simulink model "Experiment_cs"  (Simulink 8.8)
settings: Solver=ode5  StartTime=0.0  StopTime=inf  FixedStep=0.0005  RelTol=1e-3
PreLoadFcn:
  | check_NUTS_defined;
  | 
  | assignin('base',['model_closed_' bdroot],false);
InitFcn:
  | PreScanExperimentInitFcn(bdroot)
StopFcn:
  | PreScanExperimentStopFcn(bdroot)
undefined symbols (not defined in the file): DiscIntNeverNeededParam, FromPrescan, IdealSensors, psi, vd01, vd02, vd03, vd04, x, y
libraries: PreScanSimulinkLibrary x12, PreScanUsefulBlocks x8
(part 5 of 5)

== matlab function Toyota_Yaris_1/Dynamics_UserSpecified/SingleVehicle_01/Controller/CtlMainBusUnitDelayAndInit/MATLAB Function ==
  data: u input double; y output Bus: ControllerMainBus; veh_struct parameter double
function y = DelayAndInitCtlBus(u, veh_struct)
coder.extrinsic('exist')
persistent a

y0 = struct;

y0.ActuationCmdBus = struct;
y0.ActuationCmdBus.steering_cmd = 0;
y0.ActuationCmdBus.decel_cmd = 0;
y0.ActuationCmdBus.accel_cmd = 0;

y0.ArbitratedActuationReq = struct;
y0.ArbitratedActuationReq.v_des = 0;
y0.ArbitratedActuationReq.a_des = 0;
y0.ArbitratedActuationReq.psi_des = 0;
y0.ArbitratedActuationReq.dpsi_des = 0;


y0.FunctionFeatures = struct;
y0.FunctionFeatures.wpFollower = struct;
y0.FunctionFeatures.wpFollower.v_des = 0;
y0.FunctionFeatures.wpFollower.a_des = 0;
y0.FunctionFeatures.wpFollower.psi_des = 0;
y0.FunctionFeatures.wpFollower.dpsi_des = 0;


y0.situationBus = struct;
y0.situationBus.wP = struct;

y0.situationBus.wP.finalWayPoint = struct;
y0.situationBus.wP.finalWayPoint.x = 0;
y0.situationBus.wP.finalWayPoint.y = 0;
y0.situationBus.wP.finalWayPoint.z = 0;
y0.situationBus.wP.finalWayPoint.treach = 0;

y0.situationBus.wP.currentWayPoint = struct;
y0.situationBus.wP.currentWayPoint.x = 0;
y0.situationBus.wP.currentWayPoint.y = 0;
y0.situationBus.wP.currentWayPoint.z = 0;
y0.situationBus.wP.currentWayPoint.treach = 0;

y0.situationBus.wP.finalWayPointIndex = uint16(1);
y0.situationBus.wP.currentWayPointIndex = uint16(10);

%y0.situationBus.wP.wayPointArray = struct;
wPArray = struct;
wPArray.x = 0;
wPArray.y = 0;
wPArray.z = 0;
wPArray.treach = 0;
y0.situationBus.wP.wayPointArray = repmat(wPArray,100,1);


y0.situationBus.selfAwarenessBus = struct;
y0.situationBus.selfAwarenessBus.x = 0;
y0.situationBus.selfAwarenessBus.y = 0;
y0.situationBus.selfAwarenessBus.z = 0;
y0.situationBus.selfAwarenessBus.theta = 0;
y0.situationBus.selfAwarenessBus.phi = 0;
y0.situationBus.selfAwarenessBus.psi = 0;
y0.situationBus.selfAwarenessBus.u = 0;
y0.situationBus.selfAwarenessBus.v = 0;
y0.situationBus.selfAwarenessBus.w = 0;
y0.situationBus.selfAwarenessBus.dtheta = 0;
y0.situationBus.selfAwarenessBus.dphi = 0;
y0.situationBus.selfAwarenessBus.dpsi = 0;
y0.IdealSensors = struct;
y0.IdealSensors.x = 0;
y0.IdealSensors.y = 0;
y0.IdealSensors.z = 0;
y0.IdealSensors.theta = 0;
y0.IdealSensors.phi = 0;
y0.IdealSensors.psi = 0;
y0.IdealSensors.u = 0;
y0.IdealSensors.v = 0;
y0.IdealSensors.w = 0;
y0.IdealSensors.dtheta = 0;
y0.IdealSensors.dphi = 0;
y0.IdealSensors.dpsi = 0;
y0.FromPrescan = struct;
y0.FromPrescan.x = 0;
y0.FromPrescan.y = 0;
y0.FromPrescan.z = 0;
y0.FromPrescan.Rotx = 0;
y0.FromPrescan.Roty = 0;
y0.FromPrescan.Rotz = 0;
y0.FromPrescan.GPS_lat = 0;
y0.FromPrescan.GPS_long = 0;
y0.FromPrescan.u = 0;
y0.FromPrescan.GPS_alt = 0;
y0.FromPrescan.heading = 0;
y0.FromPrescan.Yaw_rate = 0;



if isempty(a)
    a = 1;
    y = y0;
    y.situationBus.wP.wayPointArray = veh_struct.initialWayPointsArray;
    y.situationBus.wP.currentWayPointIndex = veh_struct.initialCurrentWayPointIndex;
    y.situationBus.wP.finalWayPointIndex = veh_struct.initialFinalWayPointIndex;

else
    y = u;
end

== matlab function Toyota_Yaris_1/Dynamics_UserSpecified/SingleVehicle_01/Controller/FeaturedFunctions/wpFollower ==
  data: prevWpAction input Bus: wpFollower; prevSituation input Bus: situationBus; wpAction output Bus: wpFollower; veh_struct parameter double; newSituation output Bus: situationBus
function [wpAction, newSituation] = wpFollower(prevWpAction, prevSituation, veh_struct)

currentIndex = prevSituation.wP.currentWayPointIndex;
if currentIndex < 1
    currentIndex = uint16(1);
end
finalIndex = prevSituation.wP.finalWayPointIndex;

xd = prevSituation.wP.wayPointArray(currentIndex).x;
yd = prevSituation.wP.wayPointArray(currentIndex).y;
xa = prevSituation.selfAwarenessBus.x;
ya = prevSituation.selfAwarenessBus.y;
howClose = norm([xd-xa, yd-ya]);

if howClose < veh_struct.wpControl.wayPointThreshold
    if (currentIndex == finalIndex)
        currentIndex = uint16(1);
    else
        currentIndex = uint16(currentIndex + 1);
    end
end

newSituation = prevSituation;
newSituation.wP.currentWayPointIndex = uint16(currentIndex);
newSituation.wP.currentWayPoint.x = newSituation.wP.wayPointArray(currentIndex).x;
newSituation.wP.currentWayPoint.y = newSituation.wP.wayPointArray(currentIndex).y;
newSituation.wP.currentWayPoint.z = newSituation.wP.wayPointArray(currentIndex).z;
newSituation.wP.currentWayPoint.treach = newSituation.wP.wayPointArray(currentIndex).treach;

v_des_raw = min(veh_struct.wpControl.v_des_max, howClose / veh_struct.wpControl.howClose_saturate * veh_struct.wpControl.v_des_max);
psi_des_raw = atan2((yd-ya),(xd-xa));

% if psi_des_raw < 0
%     
%     dbg = 1;
%     
% end
    

v_des_old = prevWpAction.v_des;
psi_des_old = prevWpAction.psi_des;

a_des = veh_struct.wpControl.v_des_filter.lambda * (v_des_raw - v_des_old);
v_des = v_des_old + veh_struct.CONTROL_OS_SAMPLETIME * a_des;

dpsi_des = veh_struct.wpControl.psi_des_filter.lambda * (psi_des_raw - psi_des_old);
psi_des = psi_des_old + veh_struct.CONTROL_OS_SAMPLETIME * dpsi_des;
% psi_des = mod(psi_des, 2 * pi);


wpAction.v_des = v_des;
wpAction.a_des = a_des;
wpAction.psi_des = psi_des;
wpAction.dpsi_des = dpsi_des;

end

== matlab function Toyota_Yaris_1/Dynamics_UserSpecified/SingleVehicle_01/Controller/SituationalAwareness/situationAwareness ==
  data: prevSituation input Bus: situationBus; newSituation output Bus: situationBus; prescanSimData input Bus: PrescanSimData; idealSensors input Bus: VehState; veh_struct parameter double
function newSituation = calcSituationAwareness(prevSituation,prescanSimData,idealSensors, veh_struct)

newSituation = prevSituation;


newSituation.selfAwarenessBus.x = idealSensors.x;
newSituation.selfAwarenessBus.y = idealSensors.y;
newSituation.selfAwarenessBus.z = idealSensors.z;
newSituation.selfAwarenessBus.theta = idealSensors.theta;
newSituation.selfAwarenessBus.phi = idealSensors.phi;
newSituation.selfAwarenessBus.psi = idealSensors.psi;
newSituation.selfAwarenessBus.u = idealSensors.u;
newSituation.selfAwarenessBus.v = idealSensors.v;
newSituation.selfAwarenessBus.w = idealSensors.w;
newSituation.selfAwarenessBus.dtheta = idealSensors.dtheta;
newSituation.selfAwarenessBus.dphi = idealSensors.dphi;
newSituation.selfAwarenessBus.dpsi = idealSensors.dpsi;


end

== matlab function Toyota_Yaris_1/Dynamics_UserSpecified/SingleVehicle_01/Controller/StrategicArbitration/Arbitration ==
  data: FunctionFeatures input Bus: FunctionFeatures; ArbitratedReq output Bus: ArbitratedActuationReq
function ArbitratedReq = Arbitrate(FunctionFeatures)

ArbitratedReq.v_des = FunctionFeatures.wpFollower.v_des;
ArbitratedReq.a_des = FunctionFeatures.wpFollower.a_des;
ArbitratedReq.psi_des = FunctionFeatures.wpFollower.psi_des;
ArbitratedReq.dpsi_des = FunctionFeatures.wpFollower.dpsi_des;

end

== matlab function Toyota_Yaris_1/Dynamics_UserSpecified/SingleVehicle_01/VehStateBusUnitDelayAndInit/MATLAB Function ==
  data: u input double; y output Bus: VehState
function y = DelayAndInitVehState(u)
persistent a
y0 = struct;
y0.x = 1;
y0.y = 2;
y0.z = 0;
y0.theta = 0;
y0.phi = 0;
y0.psi = 0;
y0.u = 0;
y0.v = 0;
y0.w = 0;
y0.dtheta = 0;
y0.dphi = 0;
y0.dpsi = 0;

%y0 = VehState_MATLABStruct;
if isempty(a)
    a = 1;
    y = y0;
else
    y = u;
end

== matlab function Toyota_Yaris_1/Dynamics_UserSpecified/SingleVehicle_01/VehicleDynamics/KinematicVehicleModel ==
  data: u input double; delta input double; dX output double; psi input double; dY output double; dpsi output double; veh_struct parameter double
function [dX,dY,dpsi] = fcn(u,delta, psi, veh_struct)

lf = veh_struct.lf;
lr = veh_struct.lr;

% psi = unwrap(psi);
% delta = unwrap(delta);

beta = atan( lr /(lf + lr) * tan(delta));

% beta = unwrap(beta);

dX = u * cos(psi + beta);
dY = u * sin(psi + beta);
dpsi = u / lr * sin(beta);
